simulink model "AirAirCooling_Test"  (Simulink 7.7)
settings: Solver=ode45  StartTime=0.0  StopTime=10.0  RelTol=1e-3
libraries: WZM_QSS_Lib x1
settings Model: Creator=simon  LastModifiedBy=simon

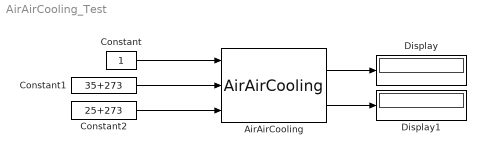
== system AirAirCooling_Test ==
  AirAirCooling : WZM_QSS_Lib/ThermalManagement/AirAirCooling  SystemSampleTime=-1  T_int_Pnts=CNC.Cooling.T_int  T_amb_Pnts=CNC.Cooling.T_ext  Qdot_extr_Pnts=CNC.Cooling.Qdot  epsilon=CNC.Cooling.epsilon
  Constant : Constant
  Constant1 : Constant  Value=35+273
  Constant2 : Constant  Value=25+273
  Display : Display
  Display1 : Display
  wires:
  Constant/1 -> AirAirCooling/1
  Constant1/1 -> AirAirCooling/2
  Constant2/1 -> AirAirCooling/3
  AirAirCooling/1 -> Display/1
  AirAirCooling/2 -> Display1/1
